simulink model "LQR_Hardware_21b"  (R2021b)
settings: Solver=ode1  StartTime=0.0  StopTime=inf  FixedStep=0.001  RelTol=1e-3  EnableMultiTasking=on
libraries: arduinolib x3, arduinosensorlib x2
settings Model: ExtModeTrigDuration=2  Creator=sokse  LastModifiedBy=sokse
settings SolverCC: AutoInsertRateTranBlk=on
settings OptimizationCC: EnhancedBackFolding=on  PassReuseOutputArgsAs=Individual arguments  ZeroExternalMemoryAtStartup=off  ZeroInternalMemoryAtStartup=off  MaxStackSize=64  OptimizeBlockOrder=speed  DifferentSizesBufferReuse=on  OptimizationCustomize=off  EfficientTunableParamExpr=on
settings DebuggingCC: ParameterTunabilityLossMsg=error  UnconnectedInputMsg=none  UnconnectedOutputMsg=none  UnconnectedLineMsg=none
settings HardwareCC: ProdBitPerInt=16  ProdBitPerPointer=16  ProdBitPerSizeT=16  ProdBitPerPtrDiffT=16  ProdLargestAtomicFloat=None  ProdWordSize=8  ProdHWDeviceType=Atmel->AVR
settings ModelReferenceCC: EnableRefExpFcnMdlSchedulingChecks=off
settings SFSimCC: MATLABDynamicMemAlloc=off
settings RTWCC: Description=Embedded Coder  SystemTargetFile=ert.tlc  HardwareBoard=Arduino Mega 2560  TemplateMakefile=ert_default_tmf  Toolchain=Arduino AVR  BuildConfiguration=Faster Runs  DLArmComputeVersion=20.02.1
settings CodeAppCC: ForceParamTrailComments=on  IgnoreCustomStorageClasses=off  OperatorAnnotations=on  SimulinkDataObjDesc=on  SFDataObjDesc=on  InsertBlockDesc=on
settings ERTTargetCC: SupportContinuousTime=on  SupportVariableSizeSignals=on  ExtModeTransport=3  ExtModeStaticAlloc=on  ExtModeStaticAllocSize=2048  ExtModeMexFile=ext_xcp  ExtModeIntrfLevel=Level2 - Open

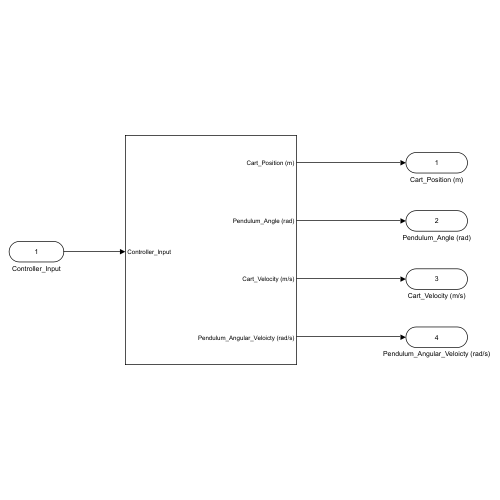
[thumbnail: Simulink's stored preview of the top-level diagram]
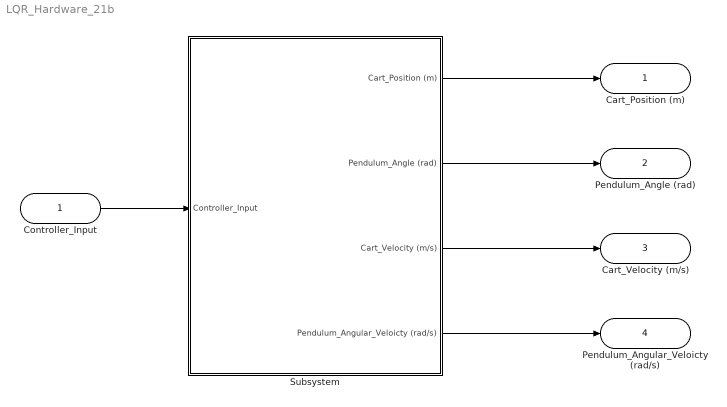
== system LQR_Hardware_21b ==
  Controller_Input : Inport
  Subsystem : Subsystem
  Cart_Position (m) : Outport
  Pendulum_Angle (rad) : Outport  Port=2
  Cart_Velocity (m/s) : Outport  Port=3
  Pendulum_Angular_Veloicty (rad/s) : Outport  Port=4
  wires:
  Controller_Input/1 -> Subsystem/1(Controller_Input)
  Subsystem/1(Cart_Position (m)) -> Cart_Position (m)/1
  Subsystem/2(Pendulum_Angle (rad)) -> Pendulum_Angle (rad)/1
  Subsystem/3(Cart_Velocity (m/s)) -> Cart_Velocity (m/s)/1
  Subsystem/4(Pendulum_Angular_Veloicty (rad/s)) -> Pendulum_Angular_Veloicty (rad/s)/1

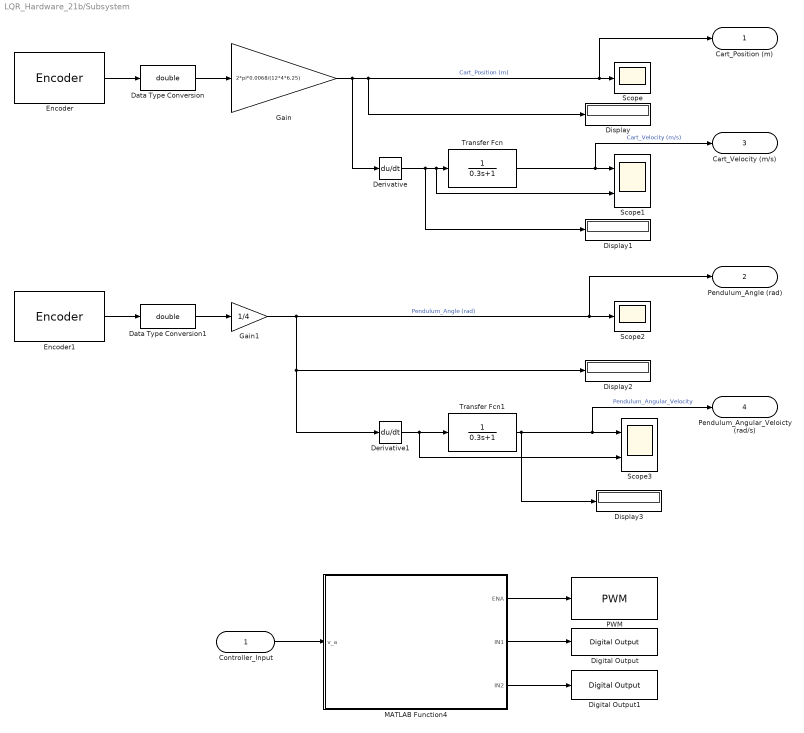
== system LQR_Hardware_21b/Subsystem ==
  Controller_Input : Inport
  Data Type Conversion : DataTypeConversion  OutDataTypeStr=double
  Data Type Conversion1 : DataTypeConversion  OutDataTypeStr=double
  Derivative : Derivative
  Derivative1 : Derivative
  Digital Output : arduinolib/Digital Output  pinNumber=5  Direction=output  blockPlatform=arduino
  Digital Output1 : arduinolib/Digital Output  pinNumber=7  Direction=output  blockPlatform=arduino
  Display{,1..3} (4 alike) : Display
  Encoder : arduinosensorlib/Encoder  InputA=2  InputB=3  Mode=No reset  SampleTime=0.01
  Encoder1 : arduinosensorlib/Encoder  InputA=20  InputB=21  Mode=No reset  SampleTime=0.01
  Gain : Gain  Gain=2*pi*0.0068/(12*4*6.25)
  Gain1 : Gain  Gain=1/4
  MATLAB Function4 : MATLAB Function  TreatAsAtomicUnit=on
  PWM : arduinolib/PWM  pinNumber=4  frequencyType=Default  desiredFrequency=490.2  achievableFrequency=490.2
  Scope : Scope
  Scope1 : Scope  NumInputPorts=2
  Scope2 : Scope
  Scope3 : Scope  NumInputPorts=2
  Transfer Fcn : TransferFcn  Denominator=[0.3 1]
  Transfer Fcn1 : TransferFcn  Denominator=[0.3 1]
  Cart_Position (m) : Outport
  Pendulum_Angle (rad) : Outport  Port=2
  Cart_Velocity (m/s) : Outport  Port=3
  Pendulum_Angular_Veloicty (rad/s) : Outport  Port=4
  wires:
  Encoder1/1 -> Data Type Conversion1/1
  MATLAB Function4/3(IN2) -> Digital Output1/1
  Gain/1 -> Derivative/1, Display/1, Cart_Position (m)/1, Scope/1  "Cart_Position (m)"
  Transfer Fcn1/1 -> Display3/1, Pendulum_Angular_Veloicty (rad/s)/1, Scope3/1  "Pendulum_Angular_Velocity"
  Data Type Conversion1/1 -> Gain1/1
  Derivative/1 -> Display1/1, Scope1/2, Transfer Fcn/1
  Derivative1/1 -> Scope3/2, Transfer Fcn1/1
  Gain1/1 -> Derivative1/1, Display2/1, Pendulum_Angle (rad)/1, Scope2/1  "Pendulum_Angle (rad)"
  Controller_Input/1 -> MATLAB Function4/1(v_a)
  Encoder/1 -> Data Type Conversion/1
  Transfer Fcn/1 -> Cart_Velocity (m/s)/1, Scope1/1  "Cart_Velocity (m/s)"
  Data Type Conversion/1 -> Gain/1
  MATLAB Function4/2(IN1) -> Digital Output/1
  MATLAB Function4/1(ENA) -> PWM/1

== matlab function LQR_Hardware_21b/Subsystem/MATLAB Function4 ==
  data: v_a input; ENA output; IN1 output; IN2 output
function [ENA,IN1,IN2] = fcn(v_a)

vmax = 12;
pwm_cal = v_a*254/vmax;

if pwm_cal > 0
   
    ENA = pwm_cal;
    IN1 = 1;
    IN2 = 0;
elseif pwm_cal < 0
   
    ENA = abs(pwm_cal);
    IN1 = 0;
    IN2 = 1;
else
    ENA = 0;
    IN1 = 0;
    IN2 = 0;
   
end
